simulink model "calcul_Mz_original"  (R2024b)
settings: Solver=FixedStepAuto  StartTime=0.0  StopTime=10.0  FixedStep=Ts  RelTol=1e-3
values from neighbouring files (symbols this model uses):
  TV = 1    [getItRunning.m]    (also in main_data_vehicle.m)
  v0 = 10    [getItRunning.m]    (also in main_data_vehicle.m)
undefined symbols (not defined in the file or in its folder): K_tab
settings Model: Creator=marti  LastModifiedBy=marti

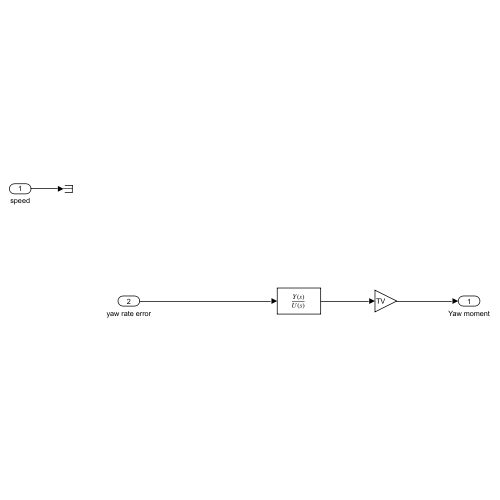
[thumbnail: Simulink's stored preview of the top-level diagram]
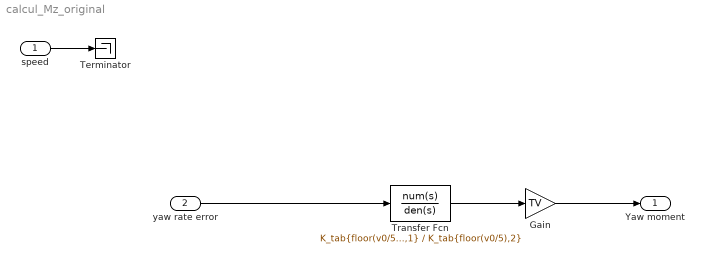
== system calcul_Mz_original ==
  speed : Inport
  yaw rate error : Inport  Port=2
  Gain : Gain  Gain=TV
  Terminator : Terminator
  Transfer Fcn : TransferFcn  Numerator=K_tab{floor(v0/5),1}  Denominator=K_tab{floor(v0/5),2}
  Yaw moment : Outport
  wires:
  speed/1 -> Terminator/1
  yaw rate error/1 -> Transfer Fcn/1
  Transfer Fcn/1 -> Gain/1
  Gain/1 -> Yaw moment/1
